simulink model "Pendulum_Calibration"  (R2024a)
settings: Solver=FixedStepAuto  StartTime=0.0  StopTime=inf  FixedStep=Tc  RelTol=1e-3  EnableMultiTasking=on
undefined symbols (not defined in the file): Tc
libraries: arduinolib x2
settings Model: ExtModeTrigDuration=2  Creator=josep  LastModifiedBy=josep
settings SolverCC: AutoInsertRateTranBlk=on
settings OptimizationCC: EnhancedBackFolding=on  PassReuseOutputArgsAs=Individual arguments  ZeroExternalMemoryAtStartup=off  ZeroInternalMemoryAtStartup=off  MaxStackSize=64  OptimizeBlockOrder=speed  DifferentSizesBufferReuse=on  OptimizationCustomize=off  EfficientTunableParamExpr=on
settings DebuggingCC: ParameterTunabilityLossMsg=error
settings HardwareCC: ProdBitPerInt=16  ProdBitPerPointer=16  ProdBitPerSizeT=16  ProdBitPerPtrDiffT=16  ProdLargestAtomicFloat=None  ProdWordSize=8  ProdHWDeviceType=Atmel->AVR
settings SFSimCC: MATLABDynamicMemAlloc=off
settings RTWCC: Description=Embedded Coder  SystemTargetFile=ert.tlc  HardwareBoard=Arduino Mega 2560  TemplateMakefile=ert_default_tmf  Toolchain=Arduino AVR  BuildConfiguration=Faster Runs
settings CodeAppCC: ForceParamTrailComments=on  IgnoreCustomStorageClasses=off  OperatorAnnotations=on  SimulinkDataObjDesc=on  SFDataObjDesc=on  InsertBlockDesc=on
settings ERTTargetCC: SupportContinuousTime=on  SupportVariableSizeSignals=on  ExtModeTransport=3  ExtModeStaticAlloc=on  ExtModeAutomaticAllocSize=off  ExtModeStaticAllocSize=2048  ExtModeMexFile=ext_xcp  ExtModeIntrfLevel=Level2 - Open

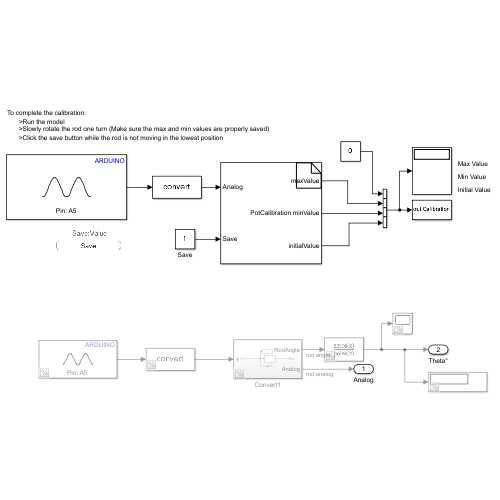
[thumbnail: Simulink's stored preview of the top-level diagram]
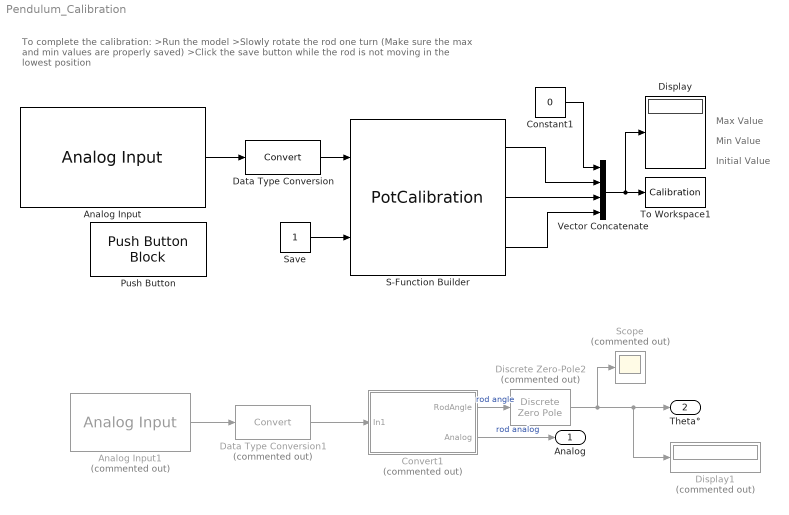
== system Pendulum_Calibration ==
  note: To complete the calibration:
      | >Run the model
      | >Slowly rotate the rod one turn (Make sure the max and min values are properly saved)
      | >Click the save button while the rod is not moving in the lowest position
  note: Min Value
  note: Initial Value
  note: Max Value
  Analog Input : arduinolib/Analog Input  pinNumber=5  ReadResultsOnly=off  ConversionTriggerSource=Software  ExternalTriggerType=uint32( 0 )  OutputDataType=uint16  EnableConversionCompleteNotify=off  EnableOuputStatus=off  SampleTime=-1  blockPlatform=arduino
  Analog Input1 : arduinolib/Analog Input  Commented=on  pinNumber=5  ReadResultsOnly=off  ConversionTriggerSource=Software  ExternalTriggerType=uint32( 0 )  OutputDataType=uint16  EnableConversionCompleteNotify=off  EnableOuputStatus=off  SampleTime=0.05  blockPlatform=arduino
  Constant1 : Constant  Value=0
  Convert1 : Subsystem  Commented=on
  Data Type Conversion : DataTypeConversion  SaturateOnIntegerOverflow=off  RndMeth=Floor
  Data Type Conversion1 : DataTypeConversion  Commented=on  SaturateOnIntegerOverflow=off  RndMeth=Floor
  Discrete Zero-Pole2 : DiscreteZeroPole  Commented=on  Zeros=[-e^(-15*Tc)]  Poles=[e^(-15*Tc)]  Gain=15*Tc/2  SampleTime=-1
  Display : Display
  Display1 : Display  Commented=on
  Push Button : PushButtonBlock  LabelPosition=Top  ButtonText=Save  OffValue=1.000000
  S-Function Builder : S-Function  InitFcn=try, set_param(gcb,'FunctionName','PotCalibration'), end  FunctionName=PotCalibration  SFunctionModules=PotCalibration_wrapper  SFunctionDeploymentMode=off  EnableBusSupport=off  mask(S-Function Builder){}
      mask help: Simulink:masks:SFunctionBuilder_MD
      mask init:
      | val = [[.9  0.75 0.75 1 1 .9 .9 1]',[1 1 0.75 0.75 .9 .9 1 .9]'];try , sys = get_param(gcb,'SfunBuilderFcnName');if isempty(sys), sys = get_param(gcb,'FunctionName'); end,catch, sys = get_param(gcb,'FunctionName'); end
      settings: CopyFcn=set_param(gcbh,'LinkStatus','none')  PreSaveFcn=try, set_param(gcb,'FunctionName','PotCalibration'), end  OpenFcn=sfunctionwizard(gcbh)
      mask Display: plot(val(:,1),val(:,2)),disp(sys), port_label('input',1,'Analog'), port_label('input',2,'Save'), port_label('output',1,'maxValue'), port_label('output',2,'minValue'), port_label('output',3,'initialValue')
  Save : Constant
  Scope : Scope  Commented=on
  To Workspace1 : ToWorkspace  VariableName=Calibration  SampleTime=-1
      settings: MaxDataPoints=1
  Vector Concatenate : Concatenate  NumInputs=4
  Analog : Outport
  Theta° : Outport  Port=2
  wires:
  S-Function Builder/3 -> Vector Concatenate/4
  Save/1 -> S-Function Builder/2
  Vector Concatenate/1 -> Display/1, To Workspace1/1
  S-Function Builder/1 -> Vector Concatenate/2
  Data Type Conversion/1 -> S-Function Builder/1
  Analog Input/1 -> Data Type Conversion/1
  Constant1/1 -> Vector Concatenate/1
  S-Function Builder/2 -> Vector Concatenate/3
  Convert1/2(Analog) -> Analog/1  "rod analog"
  Data Type Conversion1/1 -> Convert1/1(In1)
  Analog Input1/1 -> Data Type Conversion1/1
  Convert1/1(RodAngle) -> Discrete Zero-Pole2/1  "rod angle"
  Discrete Zero-Pole2/1 -> Scope/1, Display1/1, Theta°/1

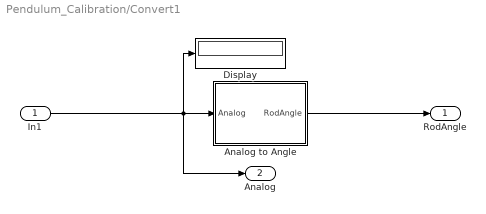
== system Pendulum_Calibration/Convert1 ==
  In1 : Inport
  Analog to Angle : Subsystem
  Display : Display
  RodAngle : Outport
  Analog : Outport  Port=2
  wires:
  In1/1 -> Analog/1, Display/1, Analog to Angle/1(Analog)
  Analog to Angle/1(RodAngle) -> RodAngle/1

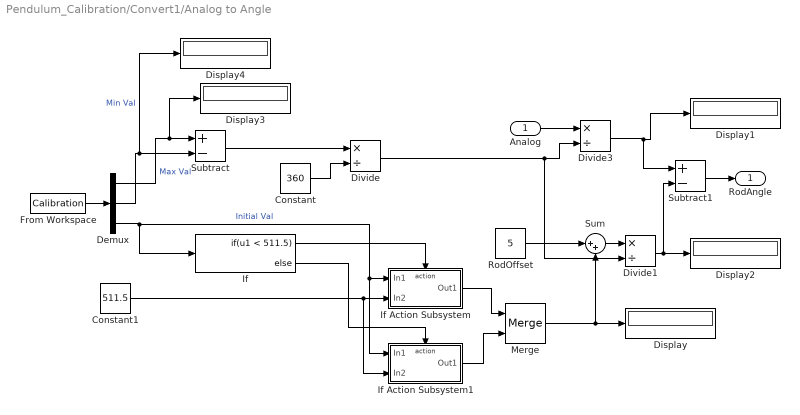
== system Pendulum_Calibration/Convert1/Analog to Angle ==
  Analog : Inport
  Constant : Constant  Value=360
  Constant1 : Constant  Value=511.5
  Demux : Demux  Outputs=3
  Display{,1..4} (5 alike) : Display
  Divide : Product  Inputs=*/
  Divide1 : Product  Inputs=*/
  Divide3 : Product  Inputs=*/
  From Workspace : FromWorkspace  VariableName=Calibration
  If : If  IfExpression=u1 < 511.5
  If Action Subsystem : Subsystem  TreatAsAtomicUnit=on
  If Action Subsystem1 : Subsystem  TreatAsAtomicUnit=on
  Merge : Merge
  RodOffset : Constant  Value=5
  Subtract : Sum  Inputs=+-
  Subtract1 : Sum  Inputs=+-
  Sum : Sum  Inputs=|++
  RodAngle : Outport
  wires:
  Demux/3 -> If/1, If Action Subsystem1/1(In1), If Action Subsystem/1(In1)  "Initial Val"
  Constant1/1 -> If Action Subsystem1/2(In2), If Action Subsystem/2(In2)
  If/1 -> If Action Subsystem/Action
  If/2 -> If Action Subsystem1/Action
  If Action Subsystem1/1(Out1) -> Merge/2
  If Action Subsystem/1(Out1) -> Merge/1
  Merge/1 -> Sum/2, Display/1
  Demux/1 -> Display3/1, Subtract/1  "Max Val"
  Demux/2 -> Display4/1, Subtract/2  "Min Val"
  Constant/1 -> Divide/2
  Subtract/1 -> Divide/1
  Divide/1 -> Divide1/2, Divide3/2
  Analog/1 -> Divide3/1
  Divide1/1 -> Display2/1, Subtract1/2
  Divide3/1 -> Display1/1, Subtract1/1
  Subtract1/1 -> RodAngle/1
  RodOffset/1 -> Sum/1
  Sum/1 -> Divide1/1
  From Workspace/1 -> Demux/1

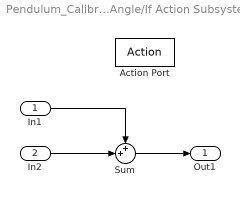
== system Pendulum_Calibration/Convert1/Analog to Angle/If Action Subsystem ==
  In1 : Inport
  In2 : Inport  Port=2
  Action Port : ActionPort  ActionPortLabel=if(u1 < 511.5)
  Sum : Sum  Inputs=++|
  Out1 : Outport  VectorParamsAs1DForOutWhenUnconnected=off
  wires:
  In1/1 -> Sum/1
  In2/1 -> Sum/2
  Sum/1 -> Out1/1

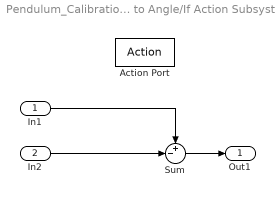
== system Pendulum_Calibration/Convert1/Analog to Angle/If Action Subsystem1 ==
  In1 : Inport
  In2 : Inport  Port=2
  Action Port : ActionPort  ActionPortLabel=else
  Sum : Sum  Inputs=+-|
  Out1 : Outport  VectorParamsAs1DForOutWhenUnconnected=off
  wires:
  In1/1 -> Sum/1
  In2/1 -> Sum/2
  Sum/1 -> Out1/1
